simulink model "double_lead_notch"  (R2021b)
settings: Solver=ode1  StartTime=0.0  StopTime=4  FixedStep=0.001  RelTol=1e-3  EnableMultiTasking=on
values from neighbouring files (symbols this model uses):
  b1 = 0.0085    [part4_prelab.m]    (also in simulation_vs_exp.m; simulation_vs_exp_3_1.m; simulation_vs_exp_3_2.m; simulation_vs_exp_3_3.m)
  b2 = 8.4745E-4    (= 0.00084745)    [part4_prelab.m]    (also in simulation_vs_exp.m; simulation_vs_exp_3_1.m; simulation_vs_exp_3_2.m; simulation_vs_exp_3_3.m)
  c = 4.2    [part4_prelab.m]    (also in simulation_vs_exp.m = 0; simulation_vs_exp_3_1.m = 0; simulation_vs_exp_3_2.m = 0; simulation_vs_exp_3_3.m = 0)
  d1 = 0.5934    [simulation_vs_exp_3_1.m]    (also in simulation_vs_exp_3_2.m; simulation_vs_exp_3_3.m)
  d2 = 0.05934    [simulation_vs_exp_3_1.m]    (also in simulation_vs_exp_3_2.m; simulation_vs_exp_3_3.m)
  k = 0.0351    [part4_prelab.m]    (also in simulation_vs_exp.m; simulation_vs_exp_3_1.m; simulation_vs_exp_3_2.m; simulation_vs_exp_3_3.m)
  kp_notch = 1/amp    [simulation_vs_exp.m]    (also in simulation_vs_exp_3_1.m; simulation_vs_exp_3_2.m; simulation_vs_exp_3_3.m)
  m1 = 2.6634E-4    (= 0.00026634)    [part4_prelab.m]    (also in simulation_vs_exp.m; simulation_vs_exp_3_1.m; simulation_vs_exp_3_2.m; simulation_vs_exp_3_3.m)
  m2 = 1.4383E-4    (= 0.00014383)    [part4_prelab.m]    (also in simulation_vs_exp.m; simulation_vs_exp_3_1.m; simulation_vs_exp_3_2.m; simulation_vs_exp_3_3.m)
  wn = 17.33    [part4_prelab.m]    (also in simulation_vs_exp.m; simulation_vs_exp_3_1.m; simulation_vs_exp_3_2.m; simulation_vs_exp_3_3.m)
  zeta = 0.2669    [part4_prelab.m]    (also in simulation_vs_exp.m; simulation_vs_exp_3_1.m; simulation_vs_exp_3_2.m; simulation_vs_exp_3_3.m)
  zeta_den = 1    [part4_prelab.m]    (also in simulation_vs_exp.m; simulation_vs_exp_3_1.m; simulation_vs_exp_3_2.m; simulation_vs_exp_3_3.m)
undefined symbols (not defined in the file or in its folder): HIL, qc_get_step_size, sgn, Ts
libraries: quarc_library x5, simulink x1
settings Model: SimulationMode=external  ExtModeTrigDuration=50000  Creator=mte360  LastModifiedBy=parth
settings SolverCC: AlgebraicLoopSolver=TrustRegion  PositivePriorityOrder=on
settings DataIOCC: LimitDataPoints=on  MaxDataPoints=100000  SaveFormat=Array  SignalLoggingSaveFormat=ModelDataLogs  ReturnWorkspaceOutputs=off
settings OptimizationCC: ExpressionDepthLimit=2147483647
settings DebuggingCC: UnderspecifiedInitializationDetection=Classic  MergeDetectMultiDrivingBlocksExec=none  SolverPrmCheckMsg=warning  FcnCallInpInsideContextMsg=warning  AllowSymbolicDim=off  StateNameClashWarn=warning  SFUnexpectedBacktrackingDiag=warning  SFNoUnconditionalDefaultTransitionDiag=warning  SFExecutionAtInitializationDiag=none  SFMachineParentedDataDiag=warning  ArithmeticOperatorsInVariantConditions=warning
settings ModelReferenceCC: PropagateSignalLabelsOutOfModel=off
settings SFSimCC: SimUseLocalCustomCode=off  CustomCodeUndefinedFunction=UseInterfaceOnly
settings RTWCC: Description=QUARC Win64 Target Using Toolchain  SystemTargetFile=quarc_win64.tlc  TemplateMakefile=quarc_default_tmf  RTWUseLocalCustomCode=off  Toolchain=QUARC win64 | nmake (64-bit Windows)  BuildConfiguration=Faster Runs
settings CodeAppCC: StateflowObjectComments=on
settings STFCustomTargetCC: ConcurrentExecutionCompliant=on  UseToolchainInfoCompliant=on  SystemTargetFile=quarc_win64.tlc
settings GRTTargetCC: TargetLangStandard=C89/C90 (ANSI)  ParMdlRefBuildCompliant=off  CompOptLevelCompliant=off  CombineOutputUpdateFcns=off  MatFileLogging=off  CPPClassGenCompliant=off  GRTInterface=on  ExtMode=on  ExtModeMexFile=quarc_comm
settings ConfigComp: CovMetricSettings=dw  CovSaveCumulativeToWorkspaceVar=on  CovSaveSingleToWorkspaceVar=on  CovExternalEMLEnable=off

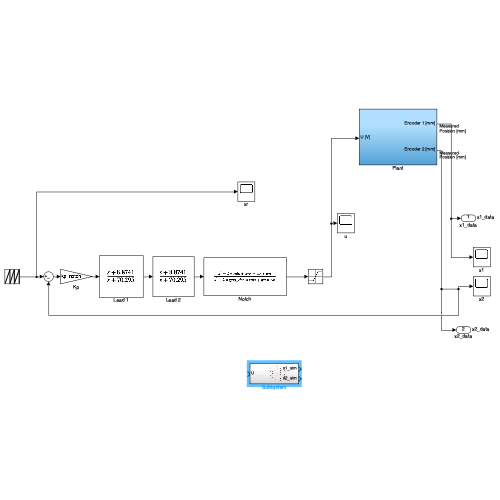
[thumbnail: Simulink's stored preview of the top-level diagram]
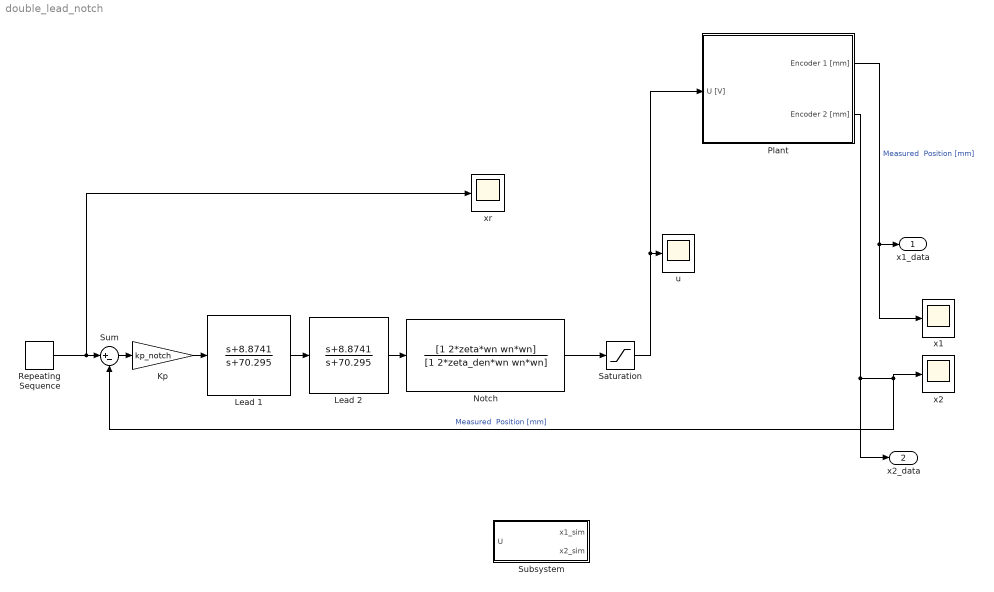
== system double_lead_notch ==
  Kp : Gain  Gain=kp_notch
  Lead 1 : TransferFcn  Numerator=[1 8.8741]  Denominator=[1 70.295]
  Lead 2 : TransferFcn  Numerator=[1 8.8741]  Denominator=[1 70.295]
  Notch : TransferFcn  Numerator=[1 2*zeta*wn wn*wn]  Denominator=[1 2*zeta_den*wn wn*wn]
  Plant : Subsystem
  Repeating Sequence : simulink/Sources/Repeating Sequence  rep_seq_t=t  rep_seq_y=s
  Saturation : Saturate  UpperLimit=8  LowerLimit=-8
  Subsystem : Subsystem
  Sum : Sum  Inputs=|+-
  u : Scope
  x1 : Scope
  x2 : Scope
  xr : Scope
  x1_data : Outport  SignalName=x1_data
  x2_data : Outport  Port=2  SignalName=x2_data
  wires:
  Repeating Sequence/1 -> xr/1, Sum/1
  Sum/1 -> Kp/1
  Plant/1(Encoder 1 [mm]) -> x1/1, x1_data/1  "Measured  Position [mm]"
  Plant/2(Encoder 2 [mm]) -> x2_data/1, x2/1, Sum/2  "Measured  Position [mm]"
  Kp/1 -> Lead 1/1
  Lead 1/1 -> Lead 2/1
  Lead 2/1 -> Notch/1
  Notch/1 -> Saturation/1
  Saturation/1 -> u/1, Plant/1(U [V])

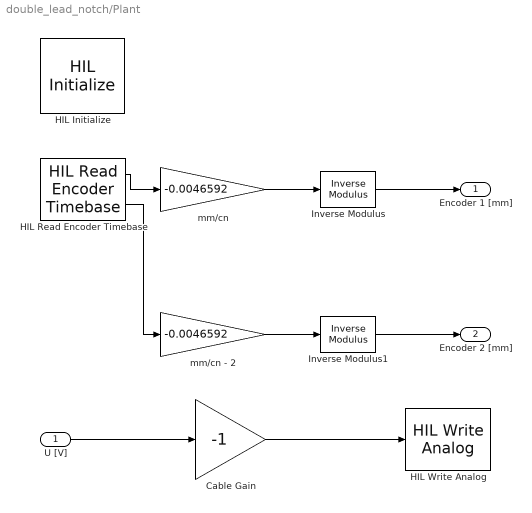
== system double_lead_notch/Plant ==
  U [V] : Inport
  Cable Gain : Gain  Gain=-1
  HIL Initialize : quarc_library/Data Acquisition/Generic/Configuration/HIL Initialize  Priority=-99  object_name=HIL-2  board_type=q2_usb  board_number=0  board_options=d0=digital;d1=digital;led=auto;update_rate=normal;decimation=1  exclusive=off  active=off  hardware_clocks=[0]  clock_modes=[]  initial_clock_frequencies=[]  set_clock_params_at_start=off  set_clock_params_at_switch_in=off  set_clock_frequencies_at_start=off  set_clock_frequencies_at_switch_in=off  analog_input_channels=[0:1]  analog_input_configurations=[]  analog_input_maximums=10  analog_input_minimums=-10  set_analog_input_params_at_start=on  set_analog_input_params_at_switch_in=off  analog_output_channels=[0:1]  analog_output_maximums=10  analog_output_minimums=-10  initial_analog_outputs=[0]  final_analog_outputs=[0]  watchdog_analog_outputs=0  set_analog_output_params_at_start=on  set_analog_output_params_at_switch_in=off  set_analog_outputs_at_start=on  set_analog_outputs_at_switch_in=off  set_analog_outputs_at_terminate=on  set_analog_outputs_at_switch_out=off  set_analog_outputs_on_watchdog=off  digital_input_channels=[]  digital_output_channels=[]  digital_output_configuration=[]  initial_digital_outputs=[1]  final_digital_outputs=[1]  watchdog_digital_outputs=[1]  set_digital_output_params_at_start=off  set_digital_output_params_at_switch_in=off  set_digital_outputs_at_start=on  set_digital_outputs_at_switch_in=off  set_digital_outputs_at_terminate=on  set_digital_outputs_at_switch_out=off  set_digital_outputs_on_watchdog=off  encoder_channels=[0:1]  quadrature=[4]  encoder_filter_frequency=[]  initial_encoder_counts=[0]  set_encoder_params_at_start=on  set_encoder_params_at_switch_in=off  set_encoder_counts_at_start=on  set_encoder_counts_at_switch_in=off  pwm_channels=[]  pwm_modes=[0]  pwm_frequency=1/0.020  pwm_configuration=[]  pwm_alignment=[]  pwm_polarity=[]  pwm_leading_deadband=[]  pwm_trailing_deadband=[]  initial_pwm_outputs=[0]  final_pwm_outputs=[0]  watchdog_pwm_outputs=[0]  set_pwm_params_at_start=on  set_pwm_params_at_switch_in=off  set_pwm_outputs_at_start=on  set_pwm_outputs_at_switch_in=off  set_pwm_outputs_at_terminate=on  set_pwm_outputs_at_switch_out=off  set_pwm_outputs_on_watchdog=off  other_output_channels=[]  initial_other_outputs=[]  final_other_outputs=[]  watchdog_other_outputs=[]  set_other_outputs_at_start=off  set_other_outputs_at_switch_in=off  set_other_outputs_at_terminate=off  set_other_outputs_at_switch_out=off  set_other_outputs_on_watchdog=off
  HIL Read Encoder Timebase : quarc_library/Data Acquisition/Generic/Timebases/HIL Read Encoder Timebase  object_name=HIL-2  clock=0  channels=[0:1]  active=on  vector_output=off  data_type_mode=Inherit via back propagation  data_type=double  overflow_mode=Error on overflow  samples_in_buffer=max(ceil(1/qc_get_step_size), 1)
  HIL Write Analog : quarc_library/Data Acquisition/Generic/Immediate I//O/HIL Write Analog  Tag=unassigned  object_name=HIL-2  channels=0  sample_time=-1  active=on  vector_input=off
  Inverse Modulus : quarc_library/Discontinuities/Inverse Modulus  modulus=65536  output_derivative=off  output_revolutions=off  max_x=Inf  min_x=-Inf
  Inverse Modulus1 : quarc_library/Discontinuities/Inverse Modulus  modulus=65536  output_derivative=off  output_revolutions=off  max_x=Inf  min_x=-Inf
  mm/cn : Gain  Gain=-0.0046592
  mm/cn - 2 : Gain  Gain=-0.0046592
  Encoder 1 [mm] : Outport
  Encoder 2 [mm] : Outport  Port=2
  wires:
  HIL Read Encoder Timebase/1 -> mm/cn/1
  U [V]/1 -> Cable Gain/1
  Cable Gain/1 -> HIL Write Analog/1
  Inverse Modulus1/1 -> Encoder 2 [mm]/1
  Inverse Modulus/1 -> Encoder 1 [mm]/1
  mm/cn - 2/1 -> Inverse Modulus1/1
  mm/cn/1 -> Inverse Modulus/1
  HIL Read Encoder Timebase/2 -> mm/cn - 2/1

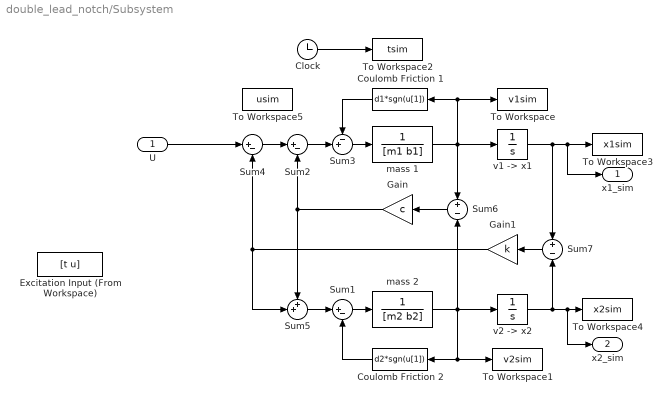
== system double_lead_notch/Subsystem ==
  U : Inport
  Clock : Clock
  Coulomb Friction 1 : Fcn  Expr=d1*sgn(u[1])
  Coulomb Friction 2 : Fcn  Expr=d2*sgn(u[1])
  Excitation Input (From Workspace) : FromWorkspace  VariableName=[t u]  SampleTime=-1  ZeroCross=off  OutputAfterFinalValue=Holding final value
  Gain : Gain  Gain=c  SaturateOnIntegerOverflow=on  OutDataTypeStr=Inherit: Same as input  ParamDataTypeStr=Inherit: Same as input
  Gain1 : Gain  Gain=k  SaturateOnIntegerOverflow=on  OutDataTypeStr=Inherit: Same as input  ParamDataTypeStr=Inherit: Same as input
  Sum1 : Sum  Inputs=|+-  SaturateOnIntegerOverflow=on
  Sum2 : Sum  Inputs=|+-  SaturateOnIntegerOverflow=on
  Sum3 : Sum  Inputs=-+|  SaturateOnIntegerOverflow=on
  Sum4 : Sum  Inputs=|+-  SaturateOnIntegerOverflow=on
  Sum5 : Sum  Inputs=++|  SaturateOnIntegerOverflow=on
  Sum6 : Sum  Inputs=+|-  SaturateOnIntegerOverflow=on
  Sum7 : Sum  Inputs=+|-  SaturateOnIntegerOverflow=on
  To Workspace : ToWorkspace  VariableName=v1sim  SampleTime=Ts
  To Workspace1 : ToWorkspace  VariableName=v2sim  SampleTime=Ts
  To Workspace2 : ToWorkspace  VariableName=tsim  SampleTime=Ts
  To Workspace3 : ToWorkspace  VariableName=x1sim  SampleTime=Ts
  To Workspace4 : ToWorkspace  VariableName=x2sim  SampleTime=Ts
  To Workspace5 : ToWorkspace  VariableName=usim  SampleTime=Ts
  mass 1 : TransferFcn  Denominator=[m1 b1]
  mass 2 : TransferFcn  Denominator=[m2 b2]
  "v1 -> x1" : Integrator
  "v2 -> x2" : Integrator
  x1_sim : Outport
  x2_sim : Outport  Port=2
  wires:
  Sum5/1 -> Sum1/1
  Coulomb Friction 1/1 -> Sum3/1
  mass 1/1 -> "v1 -> x1"/1, Sum6/1, Coulomb Friction 1/1, To Workspace/1
  Gain/1 -> Sum2/2, Sum5/1
  Sum2/1 -> Sum3/2
  Sum3/1 -> mass 1/1
  Sum4/1 -> Sum2/1
  mass 2/1 -> "v2 -> x2"/1, Sum6/2, Coulomb Friction 2/1, To Workspace1/1
  Coulomb Friction 2/1 -> Sum1/2
  Sum6/1 -> Gain/1
  Gain1/1 -> Sum4/2, Sum5/2
  Sum1/1 -> mass 2/1
  "v1 -> x1"/1 -> Sum7/1, x1_sim/1, To Workspace3/1
  Sum7/1 -> Gain1/1
  Clock/1 -> To Workspace2/1
  "v2 -> x2"/1 -> Sum7/2, x2_sim/1, To Workspace4/1
  U/1 -> Sum4/1
